simulink model "LidarLocalizationEmulation"  (R2018b)
settings: configuration reference "Active" (kept outside this file)
undefined symbols (not defined in the file): ActivateLoc_PX2, P_PX2_AMCLDelay_s, tS, tSSlow, TUMHealthStatus
libraries: simulink x1
settings Model: DataDictionary=LidarLocalizationEmulation.sldd  Creator=wischnewski  LastModifiedBy=ge34qer

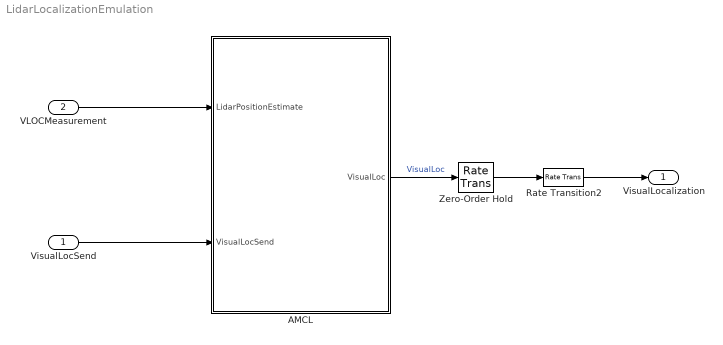
== system LidarLocalizationEmulation ==
  VisualLocSend : Inport  OutDataTypeStr=Bus: VisualLoc_Send  SampleTime=tS
  VLOCMeasurement : Inport  Port=2  OutDataTypeStr=Bus: CartPos  SampleTime=tS
  AMCL : Subsystem  SystemSampleTime=tSSlow
  Rate Transition2 : RateTransition  Deterministic=off
  Zero-Order Hold : RateTransition  OutPortSampleTime=0.04
  VisualLocalization : Outport  OutDataTypeStr=Bus: VisualLoc  SampleTime=tS  BusOutputAsStruct=on
  wires:
  AMCL/1(VisualLoc) -> Zero-Order Hold/1  "VisualLoc"
  VisualLocSend/1 -> AMCL/2(VisualLocSend)
  Zero-Order Hold/1 -> Rate Transition2/1
  Rate Transition2/1 -> VisualLocalization/1
  VLOCMeasurement/1 -> AMCL/1(LidarPositionEstimate)

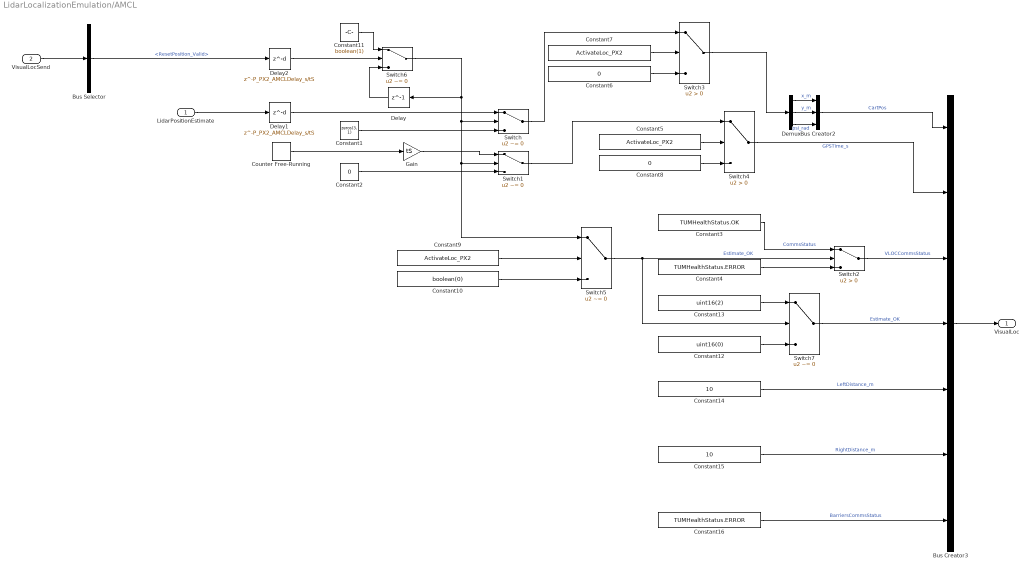
== system LidarLocalizationEmulation/AMCL ==
  LidarPositionEstimate : Inport
  VisualLocSend : Inport  Port=2
  Bus Creator2 : BusCreator  Inputs=3
  Bus Creator3 : BusCreator  Inputs=7  OutDataTypeStr=Bus: VisualLoc
  Bus Selector : BusSelector  OutputSignals=ResetPosition_Valid
  Constant1 : Constant  Value=zeros(3, 1)
  Constant10 : Constant  Value=boolean(0)
  Constant11 : Constant  Value=boolean(1)  OutDataTypeStr=boolean
  Constant12 : Constant  Value=uint16(0)
  Constant13 : Constant  Value=uint16(2)
  Constant14 : Constant  Value=10
  Constant15 : Constant  Value=10
  Constant16 : Constant  Value=TUMHealthStatus.ERROR  OutDataTypeStr=Enum: TUMHealthStatus
  Constant2 : Constant  Value=0
  Constant3 : Constant  Value=TUMHealthStatus.OK  OutDataTypeStr=Enum: TUMHealthStatus
  Constant4 : Constant  Value=TUMHealthStatus.ERROR  OutDataTypeStr=Enum: TUMHealthStatus
  Constant5 : Constant  Value=ActivateLoc_PX2
  Constant6 : Constant  Value=0
  Constant7 : Constant  Value=ActivateLoc_PX2
  Constant8 : Constant  Value=0
  Constant9 : Constant  Value=ActivateLoc_PX2
  Counter Free-Running : simulink/Sources/Counter Free-Running  NumBits=32  tsamp=tS
  Delay : Delay  DelayLength=1  InitialCondition=boolean(0)
  Delay1 : Delay  DelayLength=P_PX2_AMCLDelay_s/tS
  Delay2 : Delay  DelayLength=P_PX2_AMCLDelay_s/tS  InitialCondition=boolean(1)
  Demux : Demux  Outputs=3
  Gain : Gain  Gain=tS
  Switch{,1,5..7} (5 alike) : Switch  Criteria=u2 ~= 0
  Switch2 : Switch  Criteria=u2 > Threshold  OutDataTypeStr=Enum: TUMHealthStatus
  Switch3 : Switch  Criteria=u2 > Threshold
  Switch4 : Switch  Criteria=u2 > Threshold
  VisualLoc : Outport  OutDataTypeStr=Bus: VisualLoc
  wires:
  Demux/2 -> Bus Creator2/2  "y_m"
  Bus Creator3/1 -> VisualLoc/1
  Demux/3 -> Bus Creator2/3  "psi_rad"
  Demux/1 -> Bus Creator2/1  "x_m"
  VisualLocSend/1 -> Bus Selector/1
  Bus Creator2/1 -> Bus Creator3/1  "CartPos"
  LidarPositionEstimate/1 -> Delay1/1
  Switch6/1 -> Delay/1, Switch5/1, Switch1/2, Switch/2
  Constant1/1 -> Switch/3
  Constant2/1 -> Switch1/3
  Switch2/1 -> Bus Creator3/3  "VLOCCommsStatus"
  Constant3/1 -> Switch2/1  "CommsStatus"
  Constant4/1 -> Switch2/3
  Constant7/1 -> Switch3/2
  Constant6/1 -> Switch3/3
  Switch/1 -> Switch3/1
  Constant5/1 -> Switch4/2
  Switch1/1 -> Switch4/1
  Constant8/1 -> Switch4/3
  Constant10/1 -> Switch5/3
  Switch5/1 -> Switch7/2, Switch2/2  "Estimate_OK"
  Constant9/1 -> Switch5/2
  Switch3/1 -> Demux/1
  Switch4/1 -> Bus Creator3/2  "GPSTime_s"
  Delay1/1 -> Switch/1
  Delay/1 -> Switch6/3
  Delay2/1 -> Switch6/2
  Constant11/1 -> Switch6/1
  Bus Selector/1 -> Delay2/1  "<ResetPosition_Valid>"
  Switch7/1 -> Bus Creator3/4  "Estimate_OK"
  Constant12/1 -> Switch7/3
  Constant13/1 -> Switch7/1
  Constant14/1 -> Bus Creator3/5  "LeftDistance_m"
  Constant15/1 -> Bus Creator3/6  "RightDistance_m"
  Gain/1 -> Switch1/1
  Counter Free-Running/1 -> Gain/1
  Constant16/1 -> Bus Creator3/7  "BarriersCommsStatus"
